simulink model "Speed_ControlInverter"  (R2023b)
settings: Solver=VariableStepAuto  StartTime=0.0  StopTime=10.0  RelTol=1e-3
libraries: spsIGBTDiodeLib x6, spsDCVoltageSourceLib x1
settings Model: Creator=ADMIN  LastModifiedBy=ADMIN

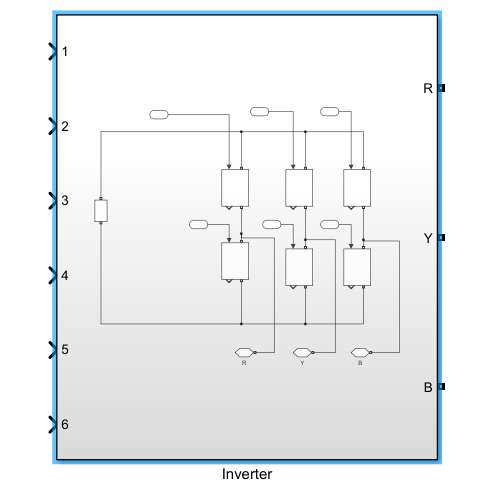
[thumbnail: Simulink's stored preview of the top-level diagram]
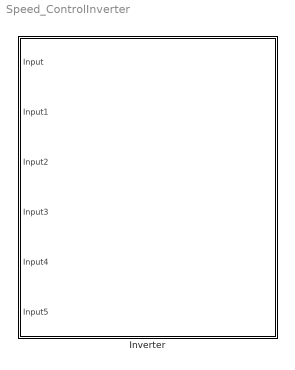
== system Speed_ControlInverter ==
  Inverter : Subsystem

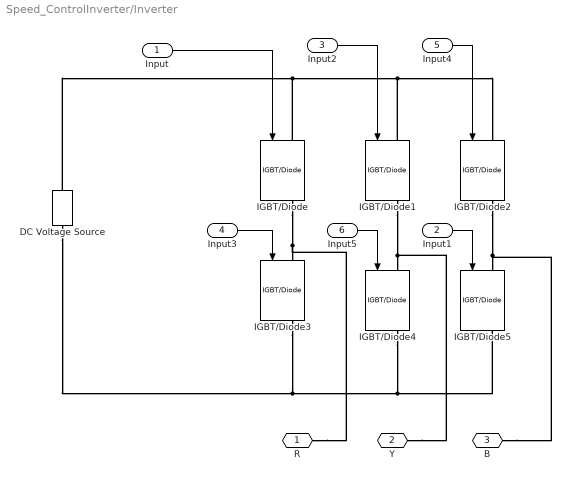
== system Speed_ControlInverter/Inverter ==
  Input : Inport
  Input1 : Inport  Port=2
  Input2 : Inport  Port=3
  Input3 : Inport  Port=4
  Input4 : Inport  Port=5
  Input5 : Inport  Port=6
  DC Voltage Source : spsDCVoltageSourceLib/DC Voltage Source  Amplitude=600  Measurements=None
  IGBT/Diode{,1..5} (6 alike) : spsIGBTDiodeLib/IGBT//Diode  Ron=1e-3  Rs=1e5  Cs=inf  Measurements=on
  R : PMIOPort  Side=Right
  Y : PMIOPort  Port=2  Side=Right
  B : PMIOPort  Port=3  Side=Right
  wires:
  Input4/1 -> IGBT/Diode2/1
  Input1/1 -> IGBT/Diode5/1
  Input5/1 -> IGBT/Diode4/1
  Input/1 -> IGBT/Diode/1
  Input3/1 -> IGBT/Diode3/1
  Input2/1 -> IGBT/Diode1/1
  connections:
  DC Voltage Source/RConn1 -- IGBT/Diode/LConn1 -- IGBT/Diode1/LConn1 -- IGBT/Diode2/LConn1
  DC Voltage Source/LConn1 -- IGBT/Diode3/RConn1 -- IGBT/Diode4/RConn1 -- IGBT/Diode5/RConn1
  IGBT/Diode1/RConn1 -- Y/RConn1 -- IGBT/Diode4/LConn1
  IGBT/Diode2/RConn1 -- B/RConn1 -- IGBT/Diode5/LConn1
  IGBT/Diode/RConn1 -- R/RConn1 -- IGBT/Diode3/LConn1
